simulink library "sensors_subsystems"  (R2023b)
settings: Solver=VariableStepAuto  StartTime=0.0  StopTime=10.0  RelTol=1e-3
undefined symbols (not defined in the file or in its folder): Environment, starTracker
libraries: $bdroot x10, matrix_library x4, vrlib x1
settings Model: Creator=brent  LastModifiedBy=brent

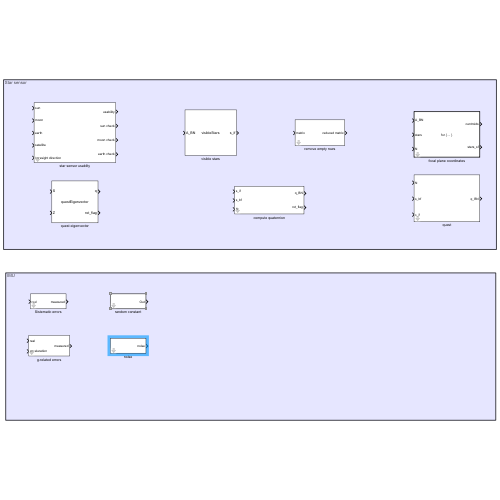
[thumbnail: Simulink's stored preview of the top-level diagram]
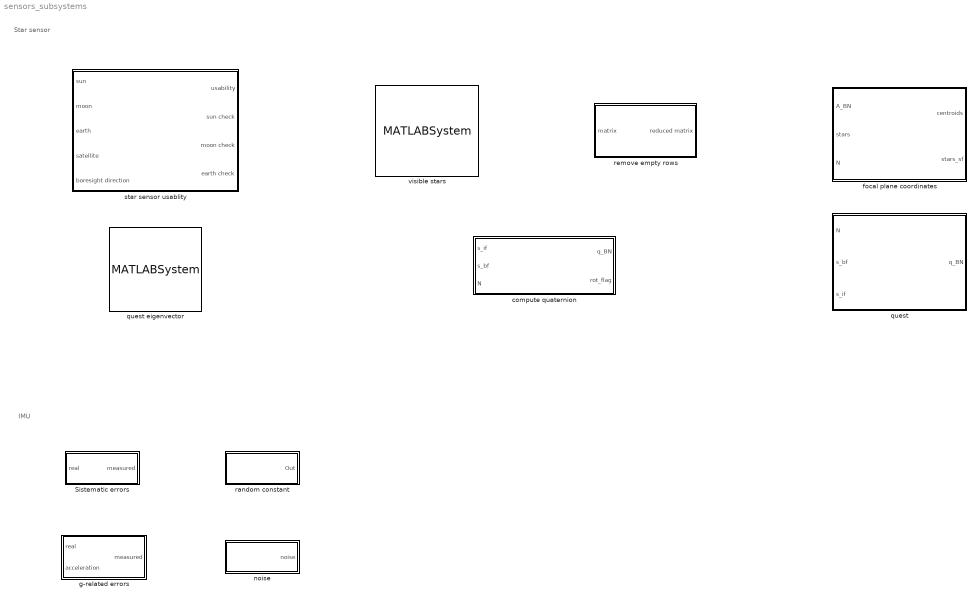
== system sensors_subsystems ==
  note: IMU
  note: Star sensor
  Sistematic errors : Subsystem  mask{data=0}
      mask prompts: data "Sensor data"
      mask DialogControl DescGroupVar Prompt: IMU deterministic errors
  compute quaternion : Subsystem  mask{starTracker=starTracker}
      mask prompts: starTracker "star tracker data"
      mask DialogControl DescGroupVar Prompt: Compute attitude quaternions using the quest method
      mask DialogControl DescTextVar Prompt: Compute the attitude quaternion given the star position in inertial and body frame and the number of visible stars
  focal plane coordinates : Subsystem  TreatAsAtomicUnit=on  mask{starTracker=starTracker, mag_seed=abs(round(rand(1)*1e4)), angle_seed=abs(round(rand(1)*1e4))}
      mask prompts: starTracker "starTracker data"; mag_seed "Magnitude noise seed"; angle_seed "Direction noise seed"
      mask DialogControl DescTextVar Prompt: Get the centroids of the star in the focal plane, given the rotation matrix from inertial to body and frame and the star vectors in inertial frame
  g-related errors : Subsystem  mask{gyro=0}
      mask prompts: gyro "Gyroscope data"
      mask DialogControl DescGroupVar Prompt: g-related errors
  noise : Subsystem  mask{data=0, white_seed=abs(round(randn(3,1)*1e4)), pink_seed=abs(round(randn(3,1)*1e4))}
      mask prompts: data "IMU data"; white_seed "White noise seeds"; pink_seed "Pink noise seeds"
      mask DialogControl DescGroupVar Prompt: White and pink noise
  quest : Subsystem
      mask DialogControl DescGroupVar Prompt: Quest
      mask DialogControl DescTextVar Prompt: Compute the quaternions to rotate a vector from inertial to body frame using the quest algorithm
  quest eigenvector : MATLABSystem  System=questEigenvector  SimulateUsing=Code generation
      mask Type: questEigenvector
      mask Display:
      | disp('questEigenvector');
      | port_label('input',1,'S');
      | port_label('input',2,'Z');
      | port_label('output',1,'q');
      | port_label('output',2,'rot_flag');
  random constant : Subsystem  mask{mean=0, dev=0}
      mask prompts: dev "Standard deviation"
      mask DialogControl DescGroupVar Prompt: Random constant
      mask DialogControl DescTextVar Prompt: Generate a random constant from a gaussian distribution with given mean and standard devition
  remove empty rows : Subsystem
      mask DialogControl DescGroupVar Prompt: Remove empty rows
      mask DialogControl ParameterGroupVar Prompt: Removes rows with only zeros from a matrix
  star sensor usablity : Subsystem  mask{R_M=Environment.Moon.radius.value, R_E=Environment.Earth.radius.value, exclusionAngle=starTracker.exclusionAngle.value, fov=starTracker.fov.value}
      mask prompts: R_M "moon radius"; R_E "earth radius"; exclusionAngle "sun exclusion angle"; fov "field of view"
      mask DialogControl DescGroupVar Prompt: Star tracker usability
      mask DialogControl DescTextVar Prompt: Check if the earth and the moon are not in the fov and that the separation with the sun is greater than the exclusion angle. If these conditions are satisfied, it returns "true", otherwise it returns "false". It also returns the status of each condition
  visible stars : MATLABSystem  System=visibleStars  starTracker=starTracker  SimulateUsing=Code generation
      mask Type: visibleStars
      mask Display:
      | disp('visibleStars');
      | port_label('input',1,'A_BN');
      | port_label('output',1,'s_if');

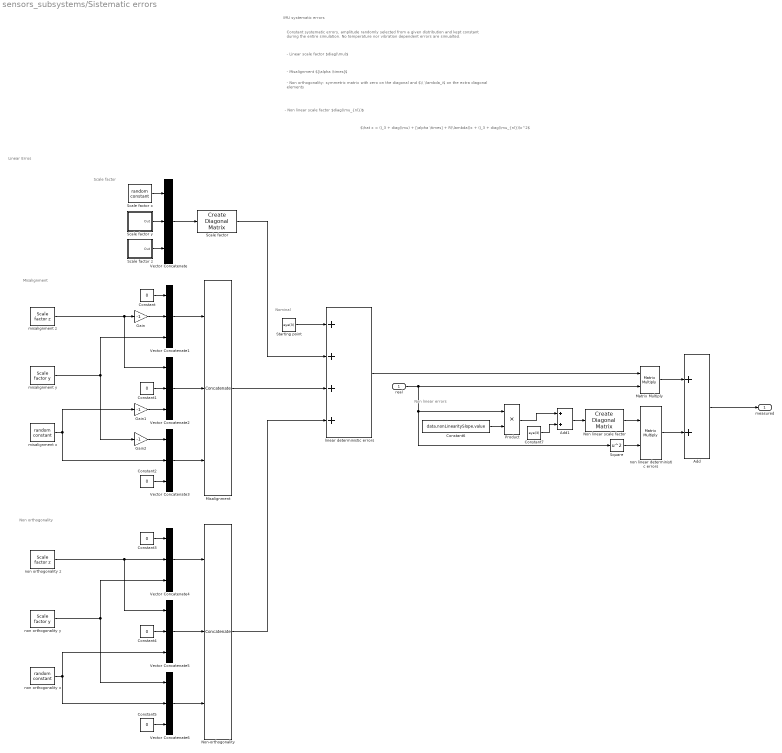
== system sensors_subsystems/Sistematic errors ==
  note: $\hat x = (I_3 + diag(\mu) + [\alpha \times] + R(\lambda))x + (I_3 + diag(\mu_{nl}))x^2$
  note: - Linear scale factor $diag(\mu)$
  note: Non orthogonality
  note: Misalignment
  note: Scale factor
  note: Nominal
  note: Linear Erros
  note: Non linear errors
  note: Constant systematic errors, amplitude randomly selected from a given distribution and kept constant during the entire simulation. No temperature nor vibration dependent errors are simualted.
  note: IMU systematic errors
  note: - Misalignment $[\alpha \times]$
  note: - Non orthogonality: symmetric matrix with zero on the diagonal and $\\ \lambda_i$ on the extra diagonal elements
  note: - Non linear scale factor $diag(\mu_{nl})$
  real : Inport
  Add : Sum
  Add1 : Sum
  Constant{,1..5} (6 alike) : Constant  Value=0
  Constant6 : Constant  Value=data.nonLinearitySlope.value
  Constant7 : Constant  Value=eye(3)
  Gain : Gain  Gain=-1
  Gain1 : Gain  Gain=-1
  Gain2 : Gain  Gain=-1
  Matrix Multiply : Product  Multiplication=Matrix(*)
  Misalignment : Concatenate  NumInputs=3  Mode=Multidimensional array  ConcatenateDimension=2
  Non linear scale factor : matrix_library/Create Diagonal Matrix
      settings: LibrarySourceBlock=|
      | simulink/Matrix
      | Operations/Create Diagonal
      | Matrix
  Non-orthogonality : Concatenate  NumInputs=3  Mode=Multidimensional array  ConcatenateDimension=2
  Product : Product
  Scale factor : matrix_library/Create Diagonal Matrix
      settings: LibrarySourceBlock=|
      | simulink/Matrix
      | Operations/Create Diagonal
      | Matrix
  Scale factor x : $bdroot/random constant  mean=data.scaleFactor.nominal  dev=data.scaleFactor.std
  Scale factor y : Subsystem  mask{mean=data.scaleFactor.nominal, dev=data.scaleFactor.std}
      mask prompts: dev "Standard deviation"
      mask DialogControl DescGroupVar Prompt: Random constant
      mask DialogControl DescTextVar Prompt: Generate a random constant from a gaussian distribution with given mean and standard devition
  Scale factor z : Subsystem  mask{mean=data.scaleFactor.nominal, dev=data.scaleFactor.std}
      mask prompts: dev "Standard deviation"
      mask DialogControl DescGroupVar Prompt: Random constant
      mask DialogControl DescTextVar Prompt: Generate a random constant from a gaussian distribution with given mean and standard devition
  Square : Math  Operator=square
  Starting point : Constant  Value=eye(3)
  Vector Concatenate{,1..6} (7 alike) : Concatenate  NumInputs=3
  linear deterministic errors : Sum  Inputs=++++
  misalignment x : $bdroot/random constant  mean=data.misalignment.nominal  dev=data.misalignment.std
  misalignment y : $bdroot/Sistematic errors/Scale factor y  mean=data.misalignment.nominal  dev=data.misalignment.std
  misalignment z : $bdroot/Sistematic errors/Scale factor z  mean=data.misalignment.nominal  dev=data.misalignment.std
  non linear deterministic errors : Product  Multiplication=Matrix(*)
  non orthogonality x : $bdroot/random constant  mean=data.nonOrthogonality.nominal  dev=data.nonOrthogonality.std
  non orthogonality y : $bdroot/Sistematic errors/Scale factor y  mean=data.nonOrthogonality.nominal  dev=data.nonOrthogonality.std
  non orthogonality z : $bdroot/Sistematic errors/Scale factor z  mean=data.nonOrthogonality.nominal  dev=data.nonOrthogonality.std
  measured : Outport
  wires:
  Vector Concatenate/1 -> Scale factor/1
  Scale factor z/1(Out) -> Vector Concatenate/3
  Scale factor x/1 -> Vector Concatenate/1
  Scale factor y/1(Out) -> Vector Concatenate/2
  Constant/1 -> Vector Concatenate1/1
  Constant1/1 -> Vector Concatenate2/2
  Constant2/1 -> Vector Concatenate3/3
  misalignment z/1 -> Vector Concatenate2/1, Gain/1
  Gain/1 -> Vector Concatenate1/2
  misalignment y/1 -> Gain2/1, Vector Concatenate1/3
  misalignment x/1 -> Gain1/1, Vector Concatenate3/2
  Gain1/1 -> Vector Concatenate2/3
  Gain2/1 -> Vector Concatenate3/1
  Vector Concatenate3/1 -> Misalignment/3
  Vector Concatenate2/1 -> Misalignment/2
  Vector Concatenate1/1 -> Misalignment/1
  non orthogonality z/1 -> Vector Concatenate4/2, Vector Concatenate5/1
  Vector Concatenate6/1 -> Non-orthogonality/3
  Constant3/1 -> Vector Concatenate4/1
  Constant5/1 -> Vector Concatenate6/3
  Constant4/1 -> Vector Concatenate5/2
  Vector Concatenate4/1 -> Non-orthogonality/1
  non orthogonality x/1 -> Vector Concatenate5/3, Vector Concatenate6/2
  non orthogonality y/1 -> Vector Concatenate6/1, Vector Concatenate4/3
  Vector Concatenate5/1 -> Non-orthogonality/2
  Non-orthogonality/1 -> linear deterministic errors/4
  Starting point/1 -> linear deterministic errors/1
  Scale factor/1 -> linear deterministic errors/2
  Misalignment/1 -> linear deterministic errors/3
  linear deterministic errors/1 -> Matrix Multiply/1
  real/1 -> Matrix Multiply/2, Product/1, Square/1
  Constant6/1 -> Product/2
  Non linear scale factor/1 -> non linear deterministic errors/1
  Square/1 -> non linear deterministic errors/2
  Matrix Multiply/1 -> Add/1
  non linear deterministic errors/1 -> Add/2
  Add/1 -> measured/1
  Add1/1 -> Non linear scale factor/1
  Product/1 -> Add1/1
  Constant7/1 -> Add1/2

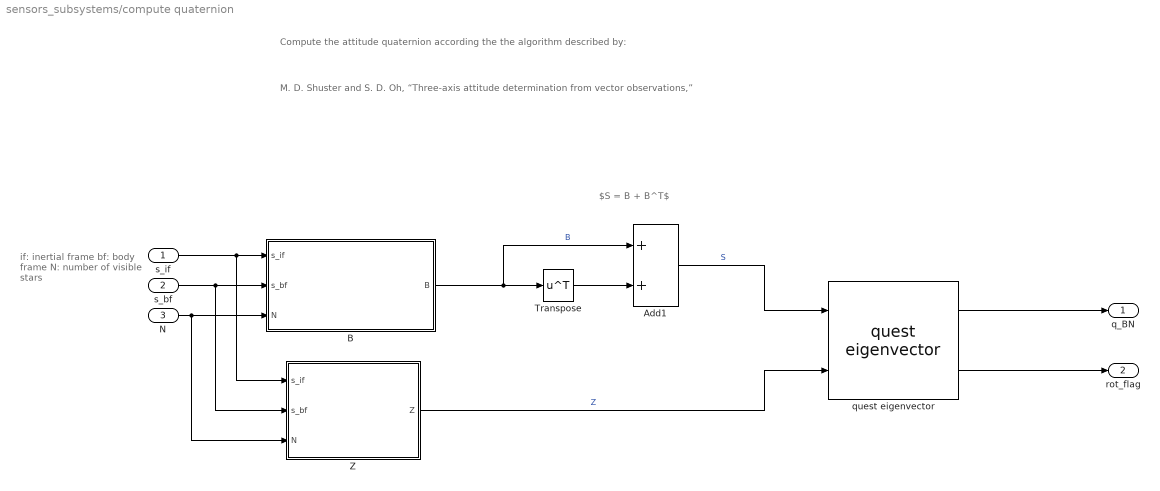
== system sensors_subsystems/compute quaternion ==
  note: if: inertial frame
      |
      | bf: body frame
      |
      | N: number of visible stars
  note: $S = B + B^T$
  note: Compute the attitude quaternion according the the algorithm described by:
  note: M. D. Shuster and S. D. Oh, “Three-axis attitude determination from vector observations,”
  s_if : Inport
  s_bf : Inport  Port=2
  N : Inport  Port=3
  Add1 : Sum
  B : Subsystem  TreatAsAtomicUnit=on
  Transpose : Math  Operator=transpose
  Z : Subsystem  TreatAsAtomicUnit=on
  quest eigenvector : $bdroot/quest eigenvector  SimulateUsing=Code generation
  q_BN : Outport
  rot_flag : Outport  Port=2
  wires:
  quest eigenvector/2 -> rot_flag/1
  quest eigenvector/1 -> q_BN/1
  Z/1(Z) -> quest eigenvector/2  "Z"
  B/1(B) -> Transpose/1, Add1/1  "B"
  Transpose/1 -> Add1/2
  Add1/1 -> quest eigenvector/1  "S"
  N/1 -> B/3(N), Z/3(N)
  s_if/1 -> B/1(s_if), Z/1(s_if)
  s_bf/1 -> B/2(s_bf), Z/2(s_bf)

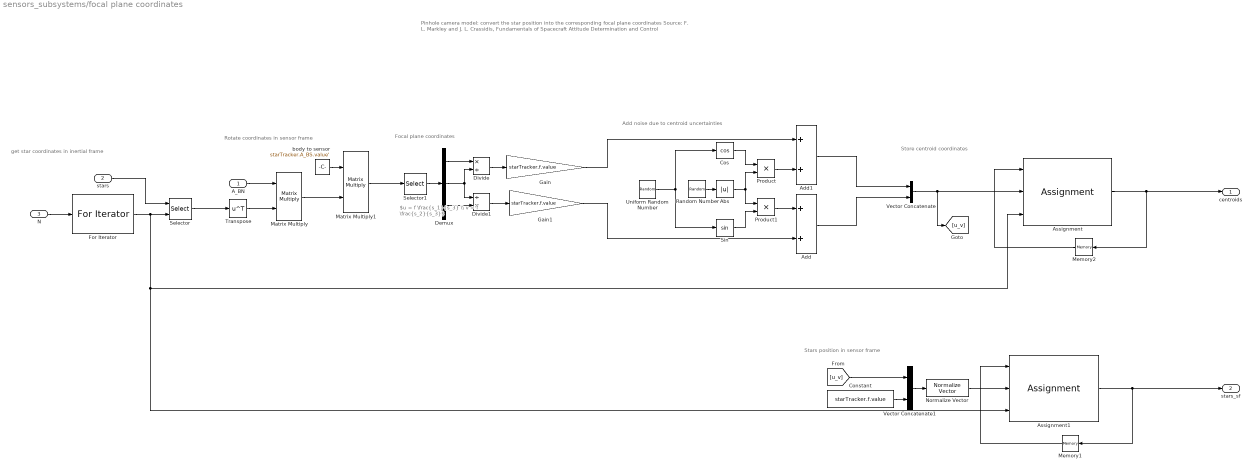
== system sensors_subsystems/focal plane coordinates ==
  note: $u = f \frac{s_1}{s_3} \\ v = f \frac{s_2}{s_3}$
  note: Stars position in sensor frame
  note: Store centroid coordinates
  note: Add noise due to centroid uncertainties
  note: Focal plane coordinates
  note: Rotate coordinates in sensor frame
  note: get star coordinates in inertial frame
  note: Pinhole camera model: convert the star position into the corresponding focal plane coordinates
      |
      | Source:
      | F. L. Markley and J. L. Crassidis, Fundamentals of Spacecraft Attitude Determination and Control
  A_BN : Inport
  stars : Inport  Port=2
  N : Inport  Port=3
  Abs : Abs  SaturateOnIntegerOverflow=off
  Add : Sum
  Add1 : Sum
  Assignment : Assignment  NumberOfDimensions=2  DiagnosticForDimensions=Warning  IndexOptions=Index vector (port),Assign all  Indices=1,1  OutputSizes=1,1
  Assignment1 : Assignment  NumberOfDimensions=2  DiagnosticForDimensions=Warning  IndexOptions=Index vector (port),Assign all  Indices=1,1  OutputSizes=1,1
  Constant : Constant  Value=starTracker.f.value
  Cos : Trigonometry  Operator=cos
  Demux : Demux  Outputs=3
  Divide : Product  Inputs=*/
  Divide1 : Product  Inputs=/*
  For Iterator : ForIterator  IterationSource=external
  Gain : Gain  Gain=starTracker.f.value
  Gain1 : Gain  Gain=starTracker.f.value
  Matrix Multiply : Product  Multiplication=Matrix(*)
  Matrix Multiply1 : Product  Multiplication=Matrix(*)
  Memory1 : Memory  InitialCondition=zeros(starTracker.maxStars.value,3)  InheritSampleTime=on
  Memory2 : Memory  InitialCondition=zeros(starTracker.maxStars.value,2)  InheritSampleTime=on
  Normalize Vector : vrlib/Utilities/Normalize Vector  maxzero=0
  Product : Product
  Product1 : Product
  Random Number : RandomNumber  Variance=(starTracker.noise.value*starTracker.pixelSize.value)^2  Seed=mag_seed  SampleTime=starTracker.sampleTime.value
  Selector : Selector  NumberOfDimensions=2  InputPortWidth=3  IndexOptions=Index vector (port),Select all  Indices=[1 3],1  OutputSizes=1,1
  Selector1 : Selector  InputPortWidth=3  IndexOptions=Index vector (dialog)  Indices=[1 3 2]  OutputSizes=1
  Sin : Trigonometry
  Transpose : Math  Operator=transpose
  Uniform Random Number : UniformRandomNumber  Minimum=0  Maximum=2*pi  Seed=angle_seed  SampleTime=starTracker.sampleTime.value
  Vector Concatenate : Concatenate  Mode=Multidimensional array  ConcatenateDimension=2
  Vector Concatenate1 : Concatenate
  body to sensor : Constant  Value=starTracker.A_BS.value'
  centroids : Outport
  stars_sf : Outport  Port=2
  wires:
  stars/1 -> Selector/1
  N/1 -> For Iterator/1
  Selector/1 -> Transpose/1
  Transpose/1 -> Matrix Multiply/2
  A_BN/1 -> Matrix Multiply/1
  Matrix Multiply/1 -> Matrix Multiply1/2
  body to sensor/1 -> Matrix Multiply1/1
  Matrix Multiply1/1 -> Selector1/1
  Selector1/1 -> Demux/1
  Demux/2 -> Divide/2, Divide1/1
  Demux/1 -> Divide/1
  Demux/3 -> Divide1/2
  Divide1/1 -> Gain1/1
  Divide/1 -> Gain/1
  Uniform Random Number/1 -> Sin/1, Cos/1
  Random Number/1 -> Abs/1
  Cos/1 -> Product/1
  Sin/1 -> Product1/2
  Abs/1 -> Product1/1, Product/2
  Product1/1 -> Add/1
  Product/1 -> Add1/2
  Gain1/1 -> Add/2
  Gain/1 -> Add1/1
  Memory2/1 -> Assignment/1
  Vector Concatenate/1 -> [u_v], Assignment/2
  Add/1 -> Vector Concatenate/2
  Add1/1 -> Vector Concatenate/1
  Assignment/1 -> centroids/1, Memory2/1
  Assignment1/1 -> stars_sf/1, Memory1/1
  For Iterator/1 -> Selector/2, Assignment1/3, Assignment/3
  Memory1/1 -> Assignment1/1
  Normalize Vector/1 -> Assignment1/2
  Vector Concatenate1/1 -> Normalize Vector/1
  Constant/1 -> Vector Concatenate1/2
  [u_v] -> Vector Concatenate1/1

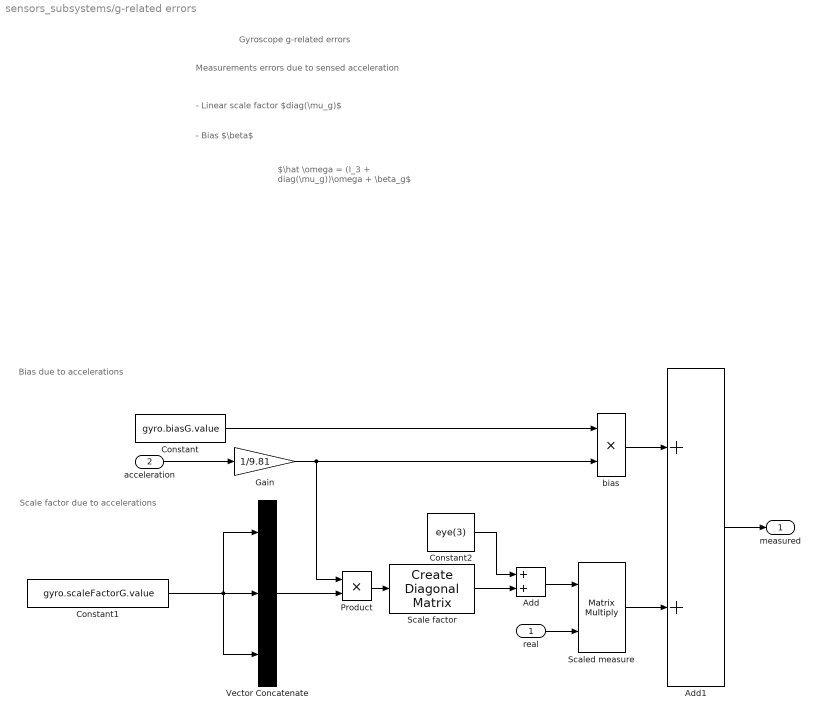
== system sensors_subsystems/g-related errors ==
  note: Scale factor due to accelerations
  note: Bias due to accelerations
  note: $\hat \omega = (I_3 + diag(\mu_g))\omega + \beta_g$
  note: Measurements errors due to sensed acceleration
  note: Gyroscope g-related errors
  note: - Linear scale factor $diag(\mu_g)$
  note: - Bias $\beta$
  real : Inport
  acceleration : Inport  Port=2
  Add : Sum
  Add1 : Sum
  Constant : Constant  Value=gyro.biasG.value
  Constant1 : Constant  Value=gyro.scaleFactorG.value
  Constant2 : Constant  Value=eye(3)
  Gain : Gain  Gain=1/9.81
  Product : Product
  Scale factor : matrix_library/Create Diagonal Matrix
      settings: LibrarySourceBlock=|
      | simulink/Matrix
      | Operations/Create Diagonal
      | Matrix
  Scaled measure : Product  Multiplication=Matrix(*)
  Vector Concatenate : Concatenate  NumInputs=3
  bias : Product
  measured : Outport
  wires:
  acceleration/1 -> Gain/1
  Constant/1 -> bias/1
  Gain/1 -> Product/1, bias/2
  Vector Concatenate/1 -> Product/2
  Constant1/1 -> Vector Concatenate/1, Vector Concatenate/3, Vector Concatenate/2
  Product/1 -> Scale factor/1
  Scale factor/1 -> Add/2
  Constant2/1 -> Add/1
  Add/1 -> Scaled measure/1
  real/1 -> Scaled measure/2
  Scaled measure/1 -> Add1/2
  bias/1 -> Add1/1
  Add1/1 -> measured/1

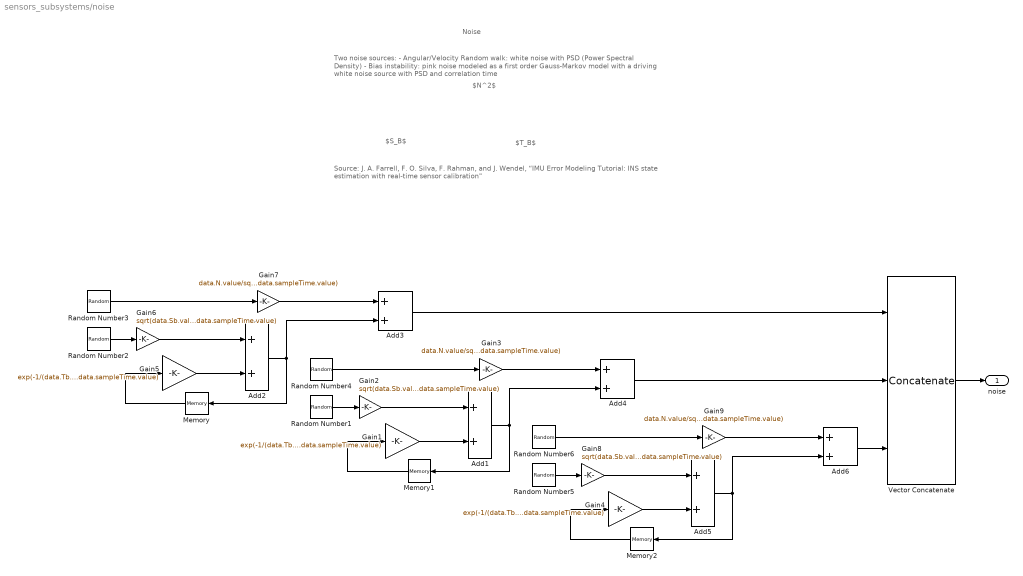
== system sensors_subsystems/noise ==
  note: $T_B$
  note: Source:
      | J. A. Farrell, F. O. Silva, F. Rahman, and J. Wendel, “IMU Error Modeling Tutorial:
      | INS state estimation with real-time sensor calibration"
  note: $S_B$
  note: $N^2$
  note: Two noise sources:
      | - Angular/Velocity Random walk: white noise with PSD (Power Spectral Density)
      |
      | - Bias instability: pink noise modeled as a first order Gauss-Markov model with a driving white noise source with PSD and correlation time
  note: Noise
  Add{1..6} (6 alike) : Sum
  Gain1 : Gain  Gain=exp(-1/(data.Tb.value)*data.sampleTime.value)
  Gain2 : Gain  Gain=sqrt(data.Sb.value*data.sampleTime.value)
  Gain3 : Gain  Gain=data.N.value/sqrt(data.sampleTime.value)
  Gain4 : Gain  Gain=exp(-1/(data.Tb.value)*data.sampleTime.value)
  Gain5 : Gain  Gain=exp(-1/(data.Tb.value)*data.sampleTime.value)
  Gain6 : Gain  Gain=sqrt(data.Sb.value*data.sampleTime.value)
  Gain7 : Gain  Gain=data.N.value/sqrt(data.sampleTime.value)
  Gain8 : Gain  Gain=sqrt(data.Sb.value*data.sampleTime.value)
  Gain9 : Gain  Gain=data.N.value/sqrt(data.sampleTime.value)
  Memory : Memory  InheritSampleTime=on
  Memory1 : Memory  InheritSampleTime=on
  Memory2 : Memory  InheritSampleTime=on
  Random Number1 : RandomNumber  Seed=pink_seed(2)  SampleTime=data.sampleTime.value
  Random Number2 : RandomNumber  Seed=pink_seed(1)  SampleTime=data.sampleTime.value
  Random Number3 : RandomNumber  Seed=white_seed(1)  SampleTime=data.sampleTime.value
  Random Number4 : RandomNumber  Seed=white_seed(2)  SampleTime=data.sampleTime.value
  Random Number5 : RandomNumber  Seed=pink_seed(3)  SampleTime=data.sampleTime.value
  Random Number6 : RandomNumber  Seed=white_seed(3)  SampleTime=data.sampleTime.value
  Vector Concatenate : Concatenate  NumInputs=3  Mode=Multidimensional array
  noise : Outport
  wires:
  Gain7/1 -> Add3/1
  Memory/1 -> Gain5/1
  Random Number2/1 -> Gain6/1
  Random Number3/1 -> Gain7/1
  Gain5/1 -> Add2/2
  Add2/1 -> Memory/1, Add3/2
  Gain6/1 -> Add2/1
  Gain1/1 -> Add1/2
  Gain3/1 -> Add4/1
  Random Number1/1 -> Gain2/1
  Memory1/1 -> Gain1/1
  Add1/1 -> Memory1/1, Add4/2
  Random Number4/1 -> Gain3/1
  Gain2/1 -> Add1/1
  Gain4/1 -> Add5/2
  Gain9/1 -> Add6/1
  Random Number5/1 -> Gain8/1
  Memory2/1 -> Gain4/1
  Add5/1 -> Memory2/1, Add6/2
  Random Number6/1 -> Gain9/1
  Gain8/1 -> Add5/1
  Add6/1 -> Vector Concatenate/3
  Add4/1 -> Vector Concatenate/2
  Add3/1 -> Vector Concatenate/1
  Vector Concatenate/1 -> noise/1

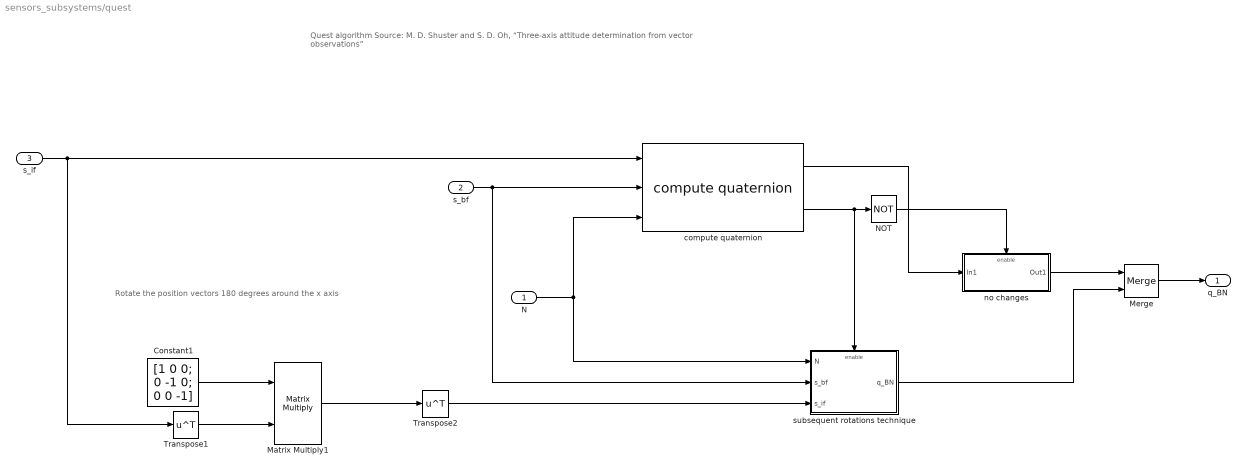
== system sensors_subsystems/quest ==
  note: Quest algorithm
      |
      | Source:
      | M. D. Shuster and S. D. Oh, “Three-axis attitude determination from vector observations”
  note: Rotate the position vectors 180 degrees around the x axis
  N : Inport
  s_bf : Inport  Port=2
  s_if : Inport  Port=3
  Constant1 : Constant  Value=[1 0 0; 0 -1 0; 0 0 -1]
  Matrix Multiply1 : Product  Multiplication=Matrix(*)
  Merge : Merge
  NOT : Logic  Operator=NOT  IconShape=distinctive  AllPortsSameDT=off  OutDataTypeStr=boolean
  Transpose1 : Math  Operator=transpose
  Transpose2 : Math  Operator=transpose
  compute quaternion : $bdroot/compute quaternion  starTracker=starTracker
  no changes : Subsystem  TreatAsAtomicUnit=on
  subsequent rotations technique : Subsystem  TreatAsAtomicUnit=on
  q_BN : Outport
  wires:
  no changes/1(Out1) -> Merge/1
  subsequent rotations technique/1(q_BN) -> Merge/2
  NOT/1 -> no changes/Enable
  compute quaternion/1 -> no changes/1(In1)
  Transpose2/1 -> subsequent rotations technique/3(s_if)
  Matrix Multiply1/1 -> Transpose2/1
  compute quaternion/2 -> NOT/1, subsequent rotations technique/Enable
  s_if/1 -> Transpose1/1, compute quaternion/1
  s_bf/1 -> compute quaternion/2, subsequent rotations technique/2(s_bf)
  Constant1/1 -> Matrix Multiply1/1
  Merge/1 -> q_BN/1
  Transpose1/1 -> Matrix Multiply1/2
  N/1 -> subsequent rotations technique/1(N), compute quaternion/3

== system sensors_subsystems/random constant ==
  Add : Sum
  Constant : Constant  Value=randn(1)
  Constant1 : Constant  Value=mean
  Gain : Gain  Gain=dev
  Out : Outport
  wires:
  Constant/1 -> Gain/1
  Gain/1 -> Add/2
  Constant1/1 -> Add/1
  Add/1 -> Out/1

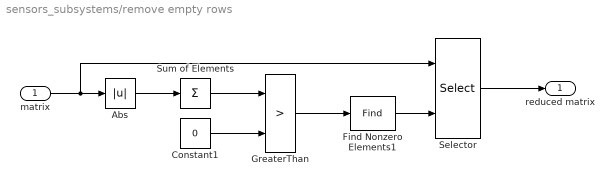
== system sensors_subsystems/remove empty rows ==
  matrix : Inport
  Abs : Abs  SaturateOnIntegerOverflow=off
  Constant1 : Constant  Value=0
  Find Nonzero Elements1 : Find  NumberOfInputDimensions=1
  GreaterThan : RelationalOperator  Operator=>  OutDataTypeStr=boolean  RndMeth=Simplest  InputSameDT=off
  Selector : Selector  NumberOfDimensions=2  InputPortWidth=3  IndexOptions=Index vector (port),Select all  Indices=[1 3],1  OutputSizes=1,1
  Sum of Elements : Sum  Inputs=+  CollapseMode=Specified dimension  CollapseDim=2
  reduced matrix : Outport
  wires:
  Abs/1 -> Sum of Elements/1
  Sum of Elements/1 -> GreaterThan/1
  matrix/1 -> Abs/1, Selector/1
  Find Nonzero Elements1/1 -> Selector/2
  Constant1/1 -> GreaterThan/2
  GreaterThan/1 -> Find Nonzero Elements1/1
  Selector/1 -> reduced matrix/1

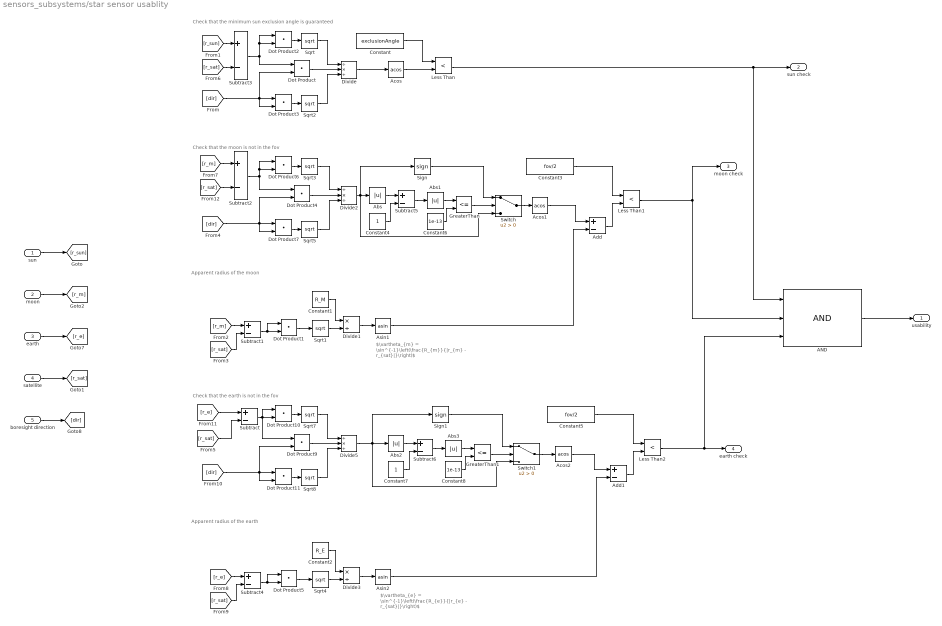
== system sensors_subsystems/star sensor usablity ==
  note: Check that the minimum sun exclusion angle is guaranteed
  note: Apparent radius of the moon
  note: $\vartheta_{m} = \sin^{-1}\left(\frac{R_{m}}{|r_{m} - r_{sat}|}\right)$
  note: Apparent radius of the earth
  note: $\vartheta_{e} = \sin^{-1}\left(\frac{R_{e}}{|r_{e} - r_{sat}|}\right)$
  note: Check that the moon is not in the fov
  note: Check that the earth is not in the fov
  sun : Inport
  moon : Inport  Port=2
  earth : Inport  Port=3
  satellite : Inport  Port=4
  boresight direction : Inport  Port=5
  AND : Logic  Inputs=3  IconShape=distinctive  AllPortsSameDT=off  OutDataTypeStr=boolean
  Abs{,1..3} (4 alike) : Abs  SaturateOnIntegerOverflow=off
  Acos : Trigonometry  Operator=acos
  Acos1 : Trigonometry  Operator=acos
  Acos2 : Trigonometry  Operator=acos
  Add : Sum  Inputs=+-
  Add1 : Sum  Inputs=+-
  Asin1 : Trigonometry  Operator=asin
  Asin2 : Trigonometry  Operator=asin
  Constant : Constant  Value=exclusionAngle
  Constant1 : Constant  Value=R_M
  Constant2 : Constant  Value=R_E
  Constant3 : Constant  Value=fov/2
  Constant4 : Constant
  Constant5 : Constant  Value=fov/2
  Constant6 : Constant  Value=1e-13
  Constant7 : Constant
  Constant8 : Constant  Value=1e-13
  Divide : Product  Inputs=/*/
  Divide1 : Product  Inputs=*/
  Divide2 : Product  Inputs=/*/
  Divide3 : Product  Inputs=*/
  Divide5 : Product  Inputs=/*/
  Dot Product{,1..7,9..11} (11 alike) : DotProduct  OutDataTypeStr=Inherit: Inherit via internal rule
  GreaterThan : RelationalOperator  Operator=<=  OutDataTypeStr=boolean  RndMeth=Simplest  InputSameDT=off
  GreaterThan1 : RelationalOperator  Operator=<=  OutDataTypeStr=boolean  RndMeth=Simplest  InputSameDT=off
  Less Than : RelationalOperator  Operator=<  OutDataTypeStr=boolean  RndMeth=Simplest  InputSameDT=off
  Less Than1 : RelationalOperator  Operator=<  OutDataTypeStr=boolean  RndMeth=Simplest  InputSameDT=off
  Less Than2 : RelationalOperator  Operator=<  OutDataTypeStr=boolean  RndMeth=Simplest  InputSameDT=off
  Sign : Signum
  Sign1 : Signum
  Sqrt{,1..5,7..8} (8 alike) : Sqrt
  Subtract{,1..6} (7 alike) : Sum  Inputs=+-
  Switch : Switch  Criteria=u2 > Threshold  SaturateOnIntegerOverflow=off  InputSameDT=off
  Switch1 : Switch  Criteria=u2 > Threshold  SaturateOnIntegerOverflow=off  InputSameDT=off
  usability : Outport
  sun check : Outport  Port=2
  moon check : Outport  Port=3
  earth check : Outport  Port=4
  wires:
  Switch1/1 -> Acos2/1
  Constant8/1 -> GreaterThan1/2
  Subtract6/1 -> Abs3/1
  Constant7/1 -> Subtract6/2
  GreaterThan1/1 -> Switch1/2
  Sign1/1 -> Switch1/1
  Abs3/1 -> GreaterThan1/1
  Divide5/1 -> Sign1/1, Abs2/1, Switch1/3
  Abs2/1 -> Subtract6/1
  Switch/1 -> Acos1/1
  Sign/1 -> Switch/1
  GreaterThan/1 -> Switch/2
  Constant6/1 -> GreaterThan/2
  Abs1/1 -> GreaterThan/1
  Subtract5/1 -> Abs1/1
  Constant4/1 -> Subtract5/2
  Abs/1 -> Subtract5/1
  Divide2/1 -> Abs/1, Switch/3, Sign/1
  Sqrt5/1 -> Divide2/3
  [r_sat] -> Subtract3/2
  Subtract3/1 -> Dot Product/1, Dot Product2/2, Dot Product2/1
  [r_sun] -> Subtract3/1
  [r_sat] -> Subtract2/2
  [r_m] -> Subtract2/1
  Subtract/1 -> Dot Product10/1, Dot Product10/2, Dot Product9/1
  [r_sat] -> Subtract/2
  Subtract2/1 -> Dot Product4/1, Dot Product6/1, Dot Product6/2
  Divide1/1 -> Asin1/1
  Sqrt1/1 -> Divide1/2
  Dot Product1/1 -> Sqrt1/1
  [r_sat] -> Subtract1/2
  [r_m] -> Subtract1/1
  Subtract1/1 -> Dot Product1/1, Dot Product1/2
  Constant1/1 -> Divide1/1
  Asin1/1 -> Add/2
  sun/1 -> [r_sun]
  satellite/1 -> [r_sat]
  moon/1 -> [r_m]
  Asin2/1 -> Add1/2
  [r_sat] -> Subtract4/2
  Constant2/1 -> Divide3/1
  Sqrt4/1 -> Divide3/2
  Dot Product5/1 -> Sqrt4/1
  [r_e] -> Subtract4/1
  Divide3/1 -> Asin2/1
  Subtract4/1 -> Dot Product5/1, Dot Product5/2
  earth/1 -> [r_e]
  boresight direction/1 -> [dir]
  Dot Product2/1 -> Sqrt/1
  [dir] -> Dot Product3/1, Dot Product/2, Dot Product3/2
  Dot Product3/1 -> Sqrt2/1
  Sqrt/1 -> Divide/1
  Dot Product/1 -> Divide/2
  Sqrt2/1 -> Divide/3
  Divide/1 -> Acos/1
  Constant/1 -> Less Than/1
  Acos/1 -> Less Than/2
  Less Than/1 -> sun check/1, AND/1
  Dot Product6/1 -> Sqrt3/1
  Sqrt3/1 -> Divide2/1
  Dot Product4/1 -> Divide2/2
  Acos1/1 -> Add/1
  [dir] -> Dot Product7/1, Dot Product4/2, Dot Product7/2
  Dot Product7/1 -> Sqrt5/1
  Add/1 -> Less Than1/2
  Constant3/1 -> Less Than1/1
  Constant5/1 -> Less Than2/1
  Add1/1 -> Less Than2/2
  Dot Product11/1 -> Sqrt8/1
  [dir] -> Dot Product11/1, Dot Product9/2, Dot Product11/2
  Acos2/1 -> Add1/1
  Sqrt7/1 -> Divide5/1
  Less Than2/1 -> earth check/1, AND/3
  Dot Product9/1 -> Divide5/2
  Dot Product10/1 -> Sqrt7/1
  [r_e] -> Subtract/1
  Sqrt8/1 -> Divide5/3
  AND/1 -> usability/1
  Less Than1/1 -> moon check/1, AND/2

== system sensors_subsystems/Sistematic errors/Scale factor y ==
  Add : Sum
  Constant : Constant  Value=randn(1)
  Constant1 : Constant  Value=mean
  Gain : Gain  Gain=dev
  Out : Outport
  wires:
  Add/1 -> Out/1
  Constant1/1 -> Add/1
  Gain/1 -> Add/2
  Constant/1 -> Gain/1

== system sensors_subsystems/Sistematic errors/Scale factor z ==
  Add : Sum
  Constant : Constant  Value=randn(1)
  Constant1 : Constant  Value=mean
  Gain : Gain  Gain=dev
  Out : Outport
  wires:
  Constant/1 -> Gain/1
  Gain/1 -> Add/2
  Constant1/1 -> Add/1
  Add/1 -> Out/1

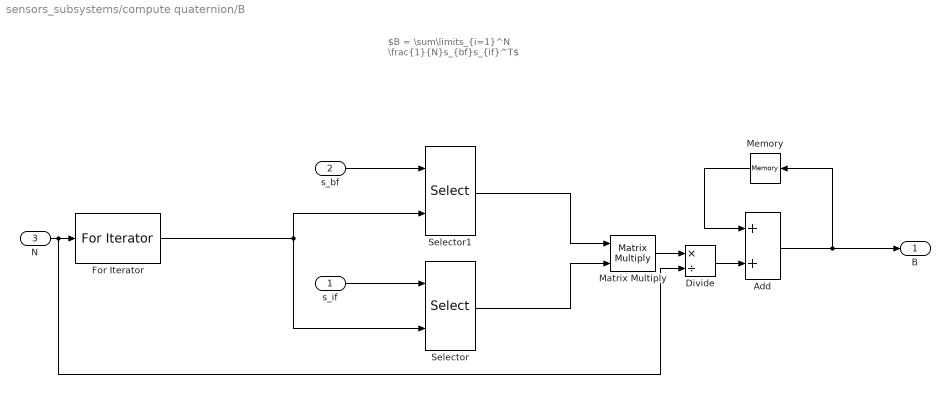
== system sensors_subsystems/compute quaternion/B ==
  note: $B = \sum\limits_{i=1}^N \frac{1}{N}s_{bf}s_{if}^T$
  s_if : Inport
  s_bf : Inport  Port=2
  N : Inport  Port=3
  Add : Sum
  Divide : Product  Inputs=*/
  For Iterator : ForIterator  ResetStates=reset  IterationSource=external
  Matrix Multiply : Product  Multiplication=Matrix(*)
  Memory : Memory  InheritSampleTime=on
  Selector : Selector  NumberOfDimensions=2  InputPortWidth=3  IndexOptions=Index vector (port),Select all  Indices=[1 3],1  OutputSizes=1,1
  Selector1 : Selector  NumberOfDimensions=2  InputPortWidth=3  IndexOptions=Select all,Index vector (port)  Indices=[1 3],1  OutputSizes=1,1
  B : Outport
  wires:
  Divide/1 -> Add/2
  Matrix Multiply/1 -> Divide/1
  Memory/1 -> Add/1
  Add/1 -> Memory/1, B/1
  Selector/1 -> Matrix Multiply/2
  Selector1/1 -> Matrix Multiply/1
  s_bf/1 -> Selector1/1
  For Iterator/1 -> Selector1/2, Selector/2
  s_if/1 -> Selector/1
  N/1 -> For Iterator/1, Divide/2

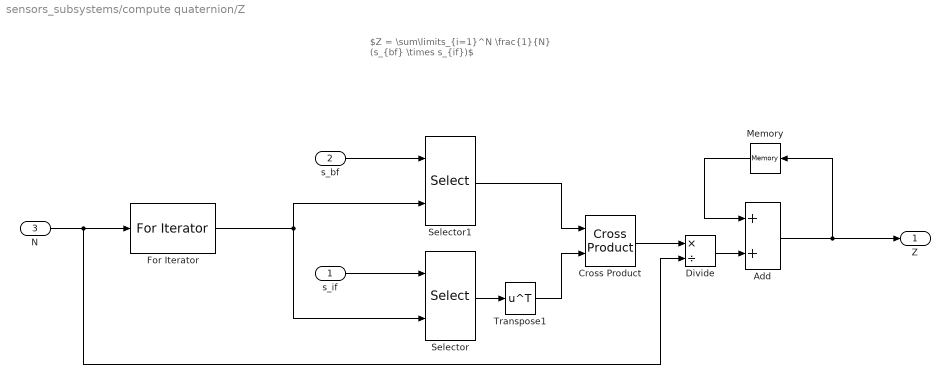
== system sensors_subsystems/compute quaternion/Z ==
  note: $Z = \sum\limits_{i=1}^N \frac{1}{N} (s_{bf} \times s_{if})$
  s_if : Inport
  s_bf : Inport  Port=2
  N : Inport  Port=3
  Add : Sum
  Cross Product : matrix_library/Cross Product
  Divide : Product  Inputs=*/
  For Iterator : ForIterator  ResetStates=reset  IterationSource=external
  Memory : Memory  InheritSampleTime=on
  Selector : Selector  NumberOfDimensions=2  InputPortWidth=3  IndexOptions=Index vector (port),Select all  Indices=[1 3],1  OutputSizes=1,1
  Selector1 : Selector  NumberOfDimensions=2  InputPortWidth=3  IndexOptions=Select all,Index vector (port)  Indices=[1 3],1  OutputSizes=1,1
  Transpose1 : Math  Operator=transpose
  Z : Outport
  wires:
  Transpose1/1 -> Cross Product/2
  N/1 -> For Iterator/1, Divide/2
  s_bf/1 -> Selector1/1
  Selector/1 -> Transpose1/1
  Selector1/1 -> Cross Product/1
  s_if/1 -> Selector/1
  Divide/1 -> Add/2
  For Iterator/1 -> Selector1/2, Selector/2
  Cross Product/1 -> Divide/1
  Memory/1 -> Add/1
  Add/1 -> Memory/1, Z/1

== system sensors_subsystems/quest/no changes ==
  In1 : Inport
  Enable : EnablePort
  Out1 : Outport
  wires:
  In1/1 -> Out1/1

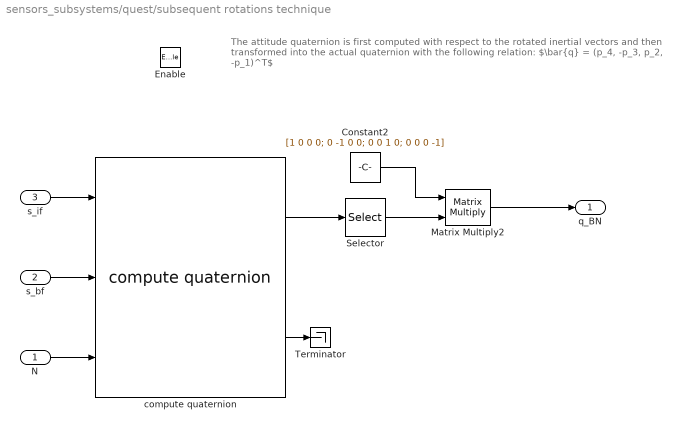
== system sensors_subsystems/quest/subsequent rotations technique ==
  note: The attitude quaternion is first computed with respect to the rotated inertial vectors and then transformed into the actual quaternion with the following relation:
      |
      | $\bar{q} = (p_4, -p_3, p_2, -p_1)^T$
  N : Inport
  s_bf : Inport  Port=2
  s_if : Inport  Port=3
  Enable : EnablePort
  Constant2 : Constant  Value=[1 0 0 0; 0 -1 0 0; 0 0 1 0; 0 0 0 -1]
  Matrix Multiply2 : Product  Multiplication=Matrix(*)
  Selector : Selector  InputPortWidth=4  IndexOptions=Index vector (dialog)  Indices=[4 3 2 1 ]  OutputSizes=1
  Terminator : Terminator
  compute quaternion : $bdroot/compute quaternion  starTracker=starTracker
  q_BN : Outport
  wires:
  s_if/1 -> compute quaternion/1
  s_bf/1 -> compute quaternion/2
  N/1 -> compute quaternion/3
  compute quaternion/2 -> Terminator/1
  compute quaternion/1 -> Selector/1
  Matrix Multiply2/1 -> q_BN/1
  Selector/1 -> Matrix Multiply2/2
  Constant2/1 -> Matrix Multiply2/1
